simulink model "pendulum"  (R2017a)
settings: Solver=VariableStepAuto  StartTime=0.0  StopTime=10.0  RelTol=1e-3
PreLoadFcn:
  | Nominal_Plant = Simulink.Variant('Mode_Plant == 1')
  | Perturbed_Plant = Simulink.Variant('Mode_Plant == 2')
  | Mode_Plant = 1
  | Linearization_Controller = Simulink.Variant('Mode_Controller == 1')
  | Integral_Controller = Simulink.Variant('Mode_Controller == 2')
  | Feedback_Linearization_Controller = Simulink.Variant('Mode_Controller == 3')
  | Mode_Controller = 1
values from neighbouring files (symbols this model uses):
  a = a0    (= 10)    [pendulum_init.m]
  a0 = 1    [SMC_continuous_integral.m]    (also in pendulum_init.m = 10)
  b = b0/2    (= 0.5)    [pendulum_init.m]
  b0 = 1    [pendulum_init.m]
  c = c0/2    (= 5)    [pendulum_init.m]
  c0 = 10    [pendulum_init.m]
  delta = pi/2    (= 1.57079632679)    [pendulum_init.m]
  delta_dot_init = 0    [pendulum_init.m]
  delta_init = 0    [pendulum_init.m]
  k1_fb = 400    [pendulum_init.m]
  k1_i = 8    [pendulum_init.m]
  k1_l = 3    [pendulum_init.m]
  k2_fb = 20    [pendulum_init.m]
  k2_i = 2    [pendulum_init.m]
  k2_l = 0.7    [pendulum_init.m]
  k3_i = 10    [pendulum_init.m]
  limit = 2    [pendulum_init.m]
  ToDeg = 180/pi    (= 57.2957795131)    [pendulum_init.m]
  w_n = 4    [pendulum_init.m]
  zeta = 1    [pendulum_init.m]
undefined symbols (not defined in the file or in its folder): sigbuilder_block
settings Model: Creator=29921  LastModifiedBy=29921

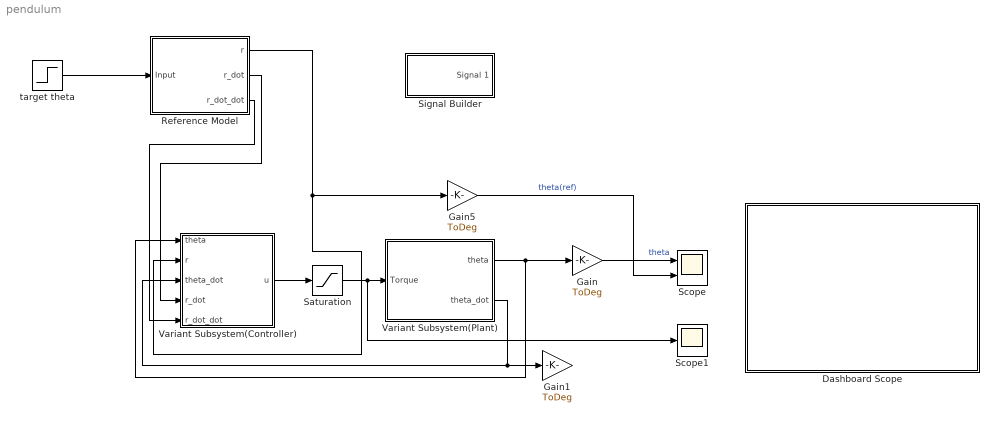
== system pendulum ==
  Dashboard Scope : Subsystem  DialogController=hmiCreateDDGDialog  IsWebBlock=on  mask(MWDashboardBlock){webBlockId=633fcfb0-8d5f-47a9-baf4-8ccff8e30ff8, webBlockType=sdiscope, ShowInitialText=on, HMISrcModelName=pendulum}
      mask prompts: webBlockId "WebBlock Id"; webBlockType "WebBlock Type"; HMISrcModelName "Source Model"
      mask help: SimulinkHMI:dialogs:HMIScopeDialogDesc
      mask Help: helpview([docroot '/mapfiles/simulink.map'], 'hmi_scope')
      mask Display:
      | if strcmp(get_param(bdroot(gcb),'BlockDiagramType'), 'library')
      |     image([(matlabroot) '/toolbox/simulink/hmi/icons/DashboardScope.png']);
      | end
  Gain : Gain  Gain=ToDeg
  Gain1 : Gain  Gain=ToDeg
  Gain5 : Gain  Gain=ToDeg
  Reference Model : Subsystem  VariantControl=Nominal_Plant
  Saturation : Saturate  UpperLimit=limit  LowerLimit=-limit
  Scope : Scope  NumInputPorts=2
  Scope1 : Scope
  Signal Builder : Subsystem  Tag=STV Subsys  LoadFcn=sigbuilder_block('load',[6 30 1012.5 446.25 ]);  StartFcn=sigbuilder_block('start');  StopFcn=sigbuilder_block('stop');  ClipboardFcn=sigbuilder_block('clipboard');  mask(Sigbuilder block){tuvar=[0:10]}
      mask help: Simulink:masks:SigbuilderBlock_MD
      mask init:
      | if ~strcmp(get_param(bdroot(gcbh),'SimulationStatus'),'stopped') tuvar = sigbuilder_block('maskInit'); end
      settings: CopyFcn=sigbuilder_block('copy');  DeleteFcn=sigbuilder_block('delete');  ModelCloseFcn=sigbuilder_block('modelClose');  PreSaveFcn=sigbuilder_block('preSave');  PauseFcn=sigbuilder_block('pause');  ContinueFcn=sigbuilder_block('continue');  NameChangeFcn=sigbuilder_block('namechange');  OpenFcn=sigbuilder_block('open',[6 30 1012.5 446.25 ]);  CloseFcn=sigbuilder_block('close');
      mask Display: plot(0, 0, 100, 100,[2, 2, 32, 32, 2], [68, 8, 8, 68, 68],[32, 2], [38, 38], [32, 19, 2],[53, 60, 44], [32, 17, 17, 2],[16, 16, 31, 31]);txt = getActiveGroup(gcbh);text(2, 100, txt,'verticalAlignment', 'top');
  Variant Subsystem(Controller) : Subsystem  Variant=on
  Variant Subsystem(Plant) : Subsystem  Variant=on
  target theta : Step  After=delta  SampleTime=0
  wires:
  Gain/1 -> Scope/1  "theta"
  Gain5/1 -> Scope/2  "theta(ref)"
  Variant Subsystem(Plant)/1(theta) -> Variant Subsystem(Controller)/1(theta), Gain/1
  Variant Subsystem(Plant)/2(theta_dot) -> Variant Subsystem(Controller)/3(theta_dot), Gain1/1
  Variant Subsystem(Controller)/1(u) -> Saturation/1
  target theta/1 -> Reference Model/1(Input)
  Reference Model/1(r) -> Variant Subsystem(Controller)/2(r), Gain5/1
  Reference Model/2(r_dot) -> Variant Subsystem(Controller)/4(r_dot)
  Reference Model/3(r_dot_dot) -> Variant Subsystem(Controller)/5(r_dot_dot)
  Saturation/1 -> Scope1/1, Variant Subsystem(Plant)/1(Torque)

== system pendulum/Dashboard Scope ==

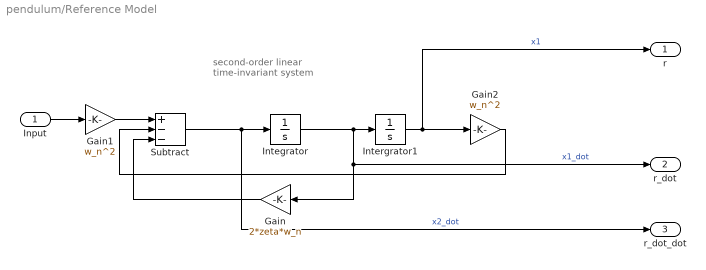
== system pendulum/Reference Model ==
  note: second-order linear time-invariant system
  Input : Inport
  Gain : Gain  Gain=2*zeta*w_n
  Gain1 : Gain  Gain=w_n^2
  Gain2 : Gain  Gain=w_n^2
  Integrator : Integrator
  Intergrator1 : Integrator
  Subtract : Sum  Inputs=+--
  r : Outport
  r_dot : Outport  Port=2
  r_dot_dot : Outport  Port=3
  wires:
  Integrator/1 -> Gain/1, r_dot/1, Intergrator1/1  "x1_dot"
  Intergrator1/1 -> Gain2/1, r/1  "x1"
  Subtract/1 -> r_dot_dot/1, Integrator/1  "x2_dot"
  Input/1 -> Gain1/1
  Gain2/1 -> Subtract/2
  Gain/1 -> Subtract/3
  Gain1/1 -> Subtract/1

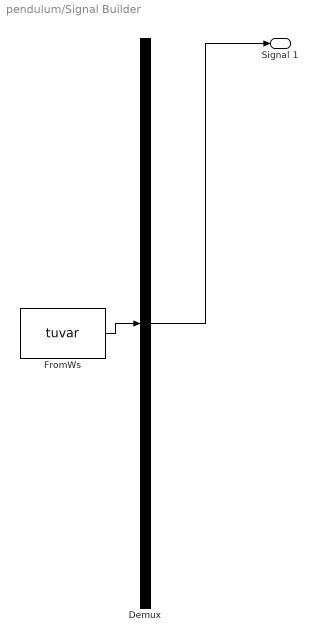
== system pendulum/Signal Builder ==
  Demux : Demux  Tag=STV Demux  Outputs=1
  FromWs : FromWorkspace  Tag=STV FromWs  VariableName=tuvar  SampleTime=0
      SigBuilderData=|
      | common.afterFinalStr = 'Extrapolate'
      | common.sampleTime = 0
      | dataSet.timeRange = [0 10]
      | dataSet.name = 'Group 1'
      | sbobj.Groups.Name = 'Group 1'
      | sbobj.Groups.Signals.Name = 'Signal 1'
      | sbobj.Groups.Signals.XData = [0 2 2 10]
      | sbobj.Groups.Signals.YData = [1.57079632679 1.57079632679 0 0]
  Signal 1 : Outport  Tag=STV Outport
  wires:
  Demux/1 -> Signal 1/1
  FromWs/1 -> Demux/1

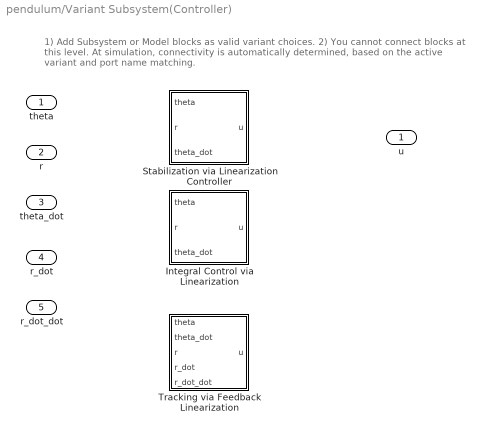
== system pendulum/Variant Subsystem(Controller) ==
  note: 1) Add Subsystem or Model blocks as valid variant choices.
      | 2) You cannot connect blocks at this level. At simulation, connectivity is automatically
      | determined, based on the active variant and port name matching.
  theta : Inport
  r : Inport  Port=2
  theta_dot : Inport  Port=3
  r_dot : Inport  Port=4
  r_dot_dot : Inport  Port=5
  Integral Control via Linearization : Subsystem  VariantControl=Integral_Controller
  Stabilization via Linearization Controller : Subsystem  VariantControl=Linearization_Controller
  Tracking via Feedback Linearization : Subsystem  VariantControl=Feedback_Linearization_Controller
  u : Outport

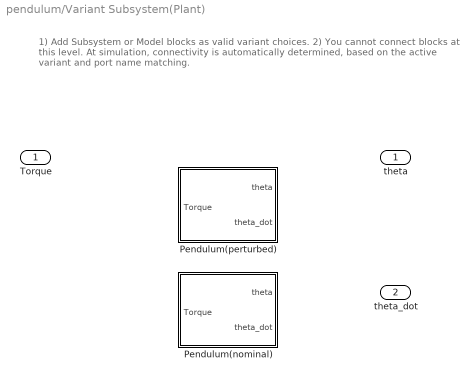
== system pendulum/Variant Subsystem(Plant) ==
  note: 1) Add Subsystem or Model blocks as valid variant choices.
      | 2) You cannot connect blocks at this level. At simulation, connectivity is automatically
      | determined, based on the active variant and port name matching.
  Torque : Inport
  Pendulum(nominal) : Subsystem  VariantControl=Nominal_Plant
  Pendulum(perturbed) : Subsystem  VariantControl=Perturbed_Plant
  theta : Outport
  theta_dot : Outport  Port=2

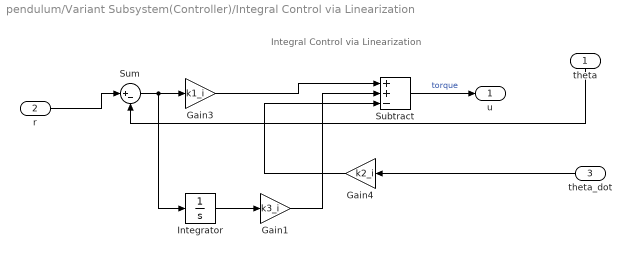
== system pendulum/Variant Subsystem(Controller)/Integral Control via Linearization ==
  note: Integral Control via Linearization
  theta : Inport
  r : Inport  Port=2
  theta_dot : Inport  Port=3
  Gain1 : Gain  Gain=k3_i
  Gain3 : Gain  Gain=k1_i
  Gain4 : Gain  Gain=k2_i
  Integrator : Integrator
  Subtract : Sum  Inputs=++-
  Sum : Sum  Inputs=|+-
  u : Outport
  wires:
  theta_dot/1 -> Gain4/1
  theta/1 -> Sum/2
  r/1 -> Sum/1
  Gain3/1 -> Subtract/1
  Gain4/1 -> Subtract/3
  Sum/1 -> Integrator/1, Gain3/1
  Subtract/1 -> u/1  "torque"
  Integrator/1 -> Gain1/1
  Gain1/1 -> Subtract/2

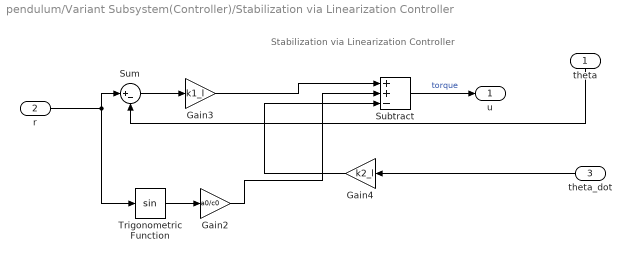
== system pendulum/Variant Subsystem(Controller)/Stabilization via Linearization Controller ==
  note: Stabilization via Linearization Controller
  theta : Inport
  r : Inport  Port=2
  theta_dot : Inport  Port=3
  Gain2 : Gain  Gain=a0/c0
  Gain3 : Gain  Gain=k1_l
  Gain4 : Gain  Gain=k2_l
  Subtract : Sum  Inputs=++-
  Sum : Sum  Inputs=|+-
  Trigonometric Function : Trigonometry
  u : Outport
  wires:
  Subtract/1 -> u/1  "torque"
  Sum/1 -> Gain3/1
  Gain4/1 -> Subtract/3
  Gain2/1 -> Subtract/2
  Trigonometric Function/1 -> Gain2/1
  Gain3/1 -> Subtract/1
  r/1 -> Sum/1, Trigonometric Function/1
  theta/1 -> Sum/2
  theta_dot/1 -> Gain4/1

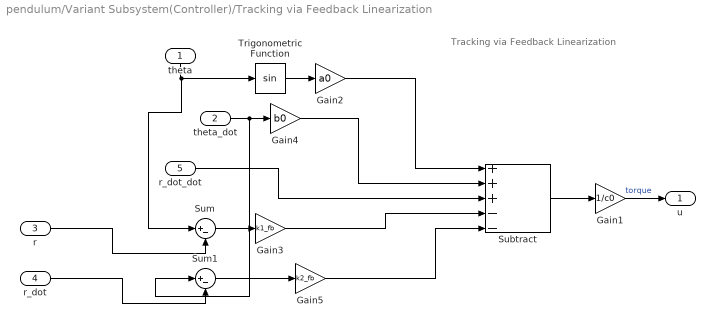
== system pendulum/Variant Subsystem(Controller)/Tracking via Feedback Linearization ==
  note: Tracking via Feedback Linearization
  theta : Inport
  theta_dot : Inport  Port=2
  r : Inport  Port=3
  r_dot : Inport  Port=4
  r_dot_dot : Inport  Port=5
  Gain1 : Gain  Gain=1/c0
  Gain2 : Gain  Gain=a0
  Gain3 : Gain  Gain=k1_fb
  Gain4 : Gain  Gain=b0
  Gain5 : Gain  Gain=k2_fb
  Subtract : Sum  Inputs=+++--
  Sum : Sum  Inputs=|+-
  Sum1 : Sum  Inputs=|+-
  Trigonometric Function : Trigonometry
  u : Outport
  wires:
  Subtract/1 -> Gain1/1
  Sum/1 -> Gain3/1
  Trigonometric Function/1 -> Gain2/1
  theta_dot/1 -> Sum1/1, Gain4/1
  Gain1/1 -> u/1  "torque"
  theta/1 -> Sum/1, Trigonometric Function/1
  Gain2/1 -> Subtract/1
  Gain4/1 -> Subtract/2
  r/1 -> Sum/2
  r_dot_dot/1 -> Subtract/3
  Gain3/1 -> Subtract/4
  r_dot/1 -> Sum1/2
  Sum1/1 -> Gain5/1
  Gain5/1 -> Subtract/5

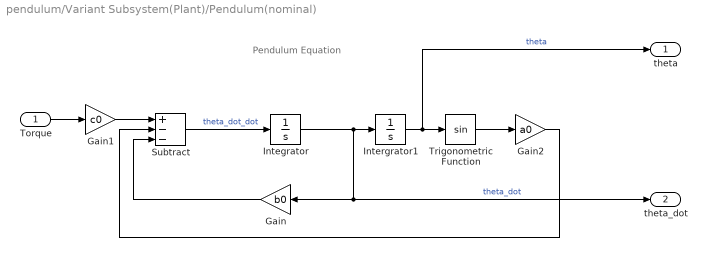
== system pendulum/Variant Subsystem(Plant)/Pendulum(nominal) ==
  note: Pendulum Equation
  Torque : Inport
  Gain : Gain  Gain=b0
  Gain1 : Gain  Gain=c0
  Gain2 : Gain  Gain=a0
  Integrator : Integrator  InitialCondition=delta_dot_init
  Intergrator1 : Integrator  InitialCondition=delta_init
  Subtract : Sum  Inputs=+--
  Trigonometric Function : Trigonometry
  theta : Outport
  theta_dot : Outport  Port=2
  wires:
  Integrator/1 -> theta_dot/1, Gain/1, Intergrator1/1  "theta_dot"
  Intergrator1/1 -> theta/1, Trigonometric Function/1  "theta"
  Subtract/1 -> Integrator/1  "theta_dot_dot"
  Torque/1 -> Gain1/1
  Trigonometric Function/1 -> Gain2/1
  Gain2/1 -> Subtract/2
  Gain/1 -> Subtract/3
  Gain1/1 -> Subtract/1

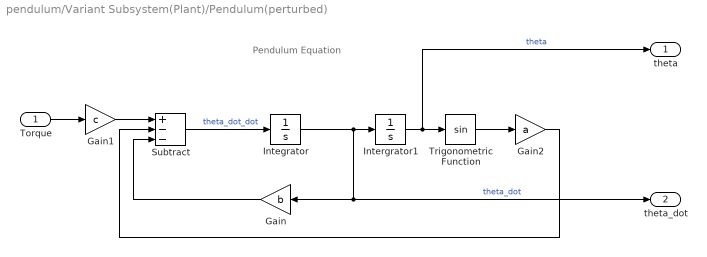
== system pendulum/Variant Subsystem(Plant)/Pendulum(perturbed) ==
  note: Pendulum Equation
  Torque : Inport
  Gain : Gain  Gain=b
  Gain1 : Gain  Gain=c
  Gain2 : Gain  Gain=a
  Integrator : Integrator  InitialCondition=delta_dot_init
  Intergrator1 : Integrator  InitialCondition=delta_init
  Subtract : Sum  Inputs=+--
  Trigonometric Function : Trigonometry
  theta : Outport
  theta_dot : Outport  Port=2
  wires:
  Integrator/1 -> theta_dot/1, Gain/1, Intergrator1/1  "theta_dot"
  Intergrator1/1 -> theta/1, Trigonometric Function/1  "theta"
  Subtract/1 -> Integrator/1  "theta_dot_dot"
  Torque/1 -> Gain1/1
  Trigonometric Function/1 -> Gain2/1
  Gain2/1 -> Subtract/2
  Gain/1 -> Subtract/3
  Gain1/1 -> Subtract/1
